simulink model "ACCMPC"  (R2023b)
settings: Solver=FixedStepDiscrete  StartTime=0.0  StopTime=1800  FixedStep=0.005  MaxStep=0.005  RelTol=1e-3  EnableMultiTasking=on
InitFcn:
  | load('DrivingCycles/WLTC.mat')
  | load('DrivingCycles/Mappa_Throttle.mat')
model workspace: external: MATLAB File C:\Users\stefa\Documents\EEPACC_MPC_CasADi_MATLAB\ACCMPC-ABO_CasADi\Init_ACCMPC_sim.m (data not in the file)
values from neighbouring files (symbols this model uses):
  OPTsettings = Settings(OPTsettings)    [Init_ACCMPC_sim.m]    (also in Main.m; Settings.m = GenerateUseCase(OPTsettings))
  V = SetVehicleParameters()    [Custom_plots.m]    (also in Init_ACCMPC_sfun.m; Init_ACCMPC_sim.m; Main.m; RunInit_ABMPC_sfun.m = SetParametersInternally())
undefined symbols (not defined in the file or in its folder): DiscIntNeverNeededParam, throttle_pedal, wheel_speed_radps, wheel_torque_Nm
libraries: slpidlib x4, simulink x1
(part 1 of 2)
settings Model: Creator=go  LastModifiedBy=stefa
settings SolverCC: ConcurrentTasks=on  AlgebraicLoopSolver=TrustRegion  PositivePriorityOrder=on  AutoInsertRateTranBlk=on
settings DataIOCC: SaveOutput=off  SaveTime=off  ReturnWorkspaceOutputs=off
settings OptimizationCC: DefaultParameterBehavior=Inlined  InlineInvariantSignals=on  EnhancedBackFolding=on  PassReuseOutputArgsAs=Individual arguments  StateBitsets=on  DataBitsets=on  ZeroExternalMemoryAtStartup=off  ZeroInternalMemoryAtStartup=off  NoFixptDivByZeroProtection=on  LifeSpan=1  OptimizeBlockOrder=speed  DifferentSizesBufferReuse=on  EfficientTunableParamExpr=on
settings DebuggingCC: TasksWithSamePriorityMsg=none  ParameterTunabilityLossMsg=error  UnconnectedInputMsg=warning  UnconnectedOutputMsg=warning  UnconnectedLineMsg=warning  ArithmeticOperatorsInVariantConditions=warning
settings HardwareCC: ProdBitPerPointer=32  ProdBitPerSizeT=32  ProdBitPerPtrDiffT=32  ProdLargestAtomicFloat=None  ProdIntDivRoundTo=Floor  ProdWordSize=32  ProdHWDeviceType=Generic->Custom
settings ModelReferenceCC: EnableRefExpFcnMdlSchedulingChecks=on
settings SFSimCC: SimUseLocalCustomCode=off  CustomCodeUndefinedFunction=UseInterfaceOnly  SimTargetLang=C++
settings RTWCC: Description=Embedded Coder  SystemTargetFile=ert.tlc  TLCOptions=-p0  GenCodeOnly=on  TemplateMakefile=ert_default_tmf  GenerateReport=on  RTWVerbose=off  RTWUseLocalCustomCode=off  Toolchain=Simulink Real-Time Toolchain  BuildConfiguration=Faster Runs  IncludeHyperlinkInReport=on  LaunchReport=on  CodeExecutionProfiling=on  TargetLang=C++  DLArmComputeVersion=19.05
settings CodeAppCC: ForceParamTrailComments=on  IgnoreCustomStorageClasses=off  MaxIdLength=95  OperatorAnnotations=on  SimulinkDataObjDesc=on  SFDataObjDesc=on  CustomSymbolStrGlobalVar=rt$N$M  CustomSymbolStrType=$N$M  CustomSymbolStrFcn=$N$M$F  CustomSymbolStrMacro=$N$M  InsertBlockDesc=on
settings ERTTargetCC: TargetLangStandard=C++03 (ISO)  CodeReplacementLibrary=ISO_C  GenerateSampleERTMain=on  SuppressErrorStatus=on  SupportAbsoluteTime=off  PurelyIntegerCode=on  SupportNonFinite=off  SupportComplex=off  InlinedParameterPlacement=NonHierarchical  RootIOFormat=Structure reference  ERTCustomFileTemplate=example_file_process.tlc

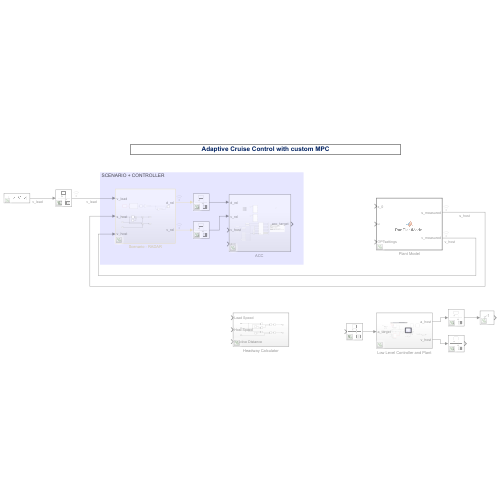
[thumbnail: Simulink's stored preview of the top-level diagram]
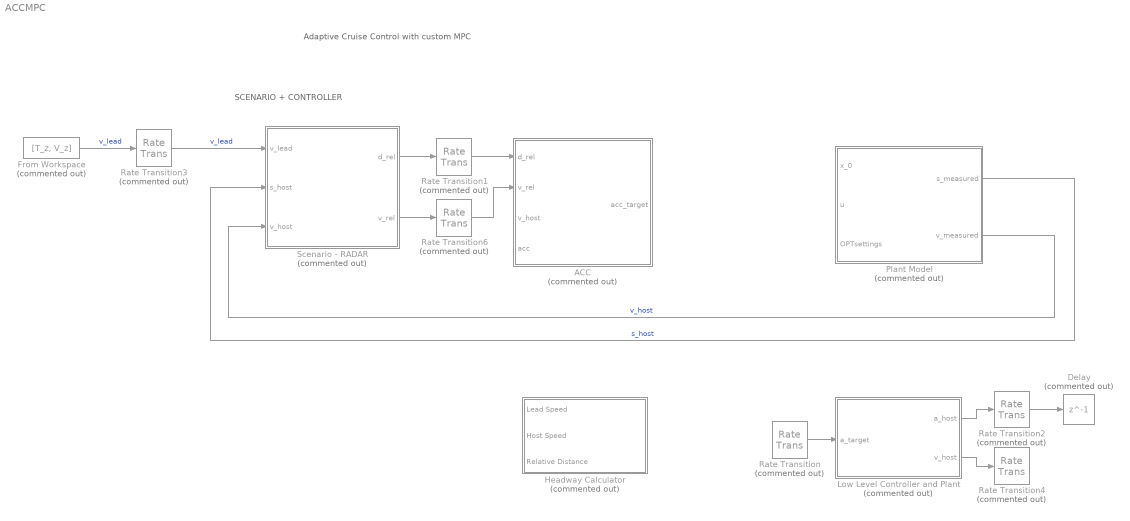
== system ACCMPC ==
  note: SCENARIO + CONTROLLER
  note: Adaptive Cruise Control with custom MPC
  "ACC " : Subsystem  Commented=on
  Delay : Delay  Commented=on  DelayLength=1
  From Workspace : FromWorkspace  Commented=on  VariableName=[T_z, V_z]  OutDataTypeStr=double  SampleTime=1
  Headway Calculator : Subsystem  Commented=on
  Low Level Controller and Plant : Subsystem  Commented=on
  Plant Model : MATLAB Function  Commented=on  TreatAsAtomicUnit=on
  Rate Transition : RateTransition  Commented=on  Integrity=off  Deterministic=off  OutPortSampleTime=0.005
  Rate Transition1 : RateTransition  Commented=on  OutPortSampleTime=0.2
  Rate Transition2 : RateTransition  Commented=on  Integrity=off  Deterministic=off  OutPortSampleTime=0.2
  Rate Transition3 : RateTransition  Commented=on  Integrity=off
  Rate Transition4 : RateTransition  Commented=on  Integrity=off  Deterministic=off  OutPortSampleTime=0.2
  Rate Transition6 : RateTransition  Commented=on  OutPortSampleTime=0.2
  Scenario - RADAR : Subsystem  Commented=on
  wires:
  Scenario - RADAR/1(d_rel) -> Rate Transition1/1
  Scenario - RADAR/2(v_rel) -> Rate Transition6/1
  Rate Transition/1 -> Low Level Controller and Plant/1(a_target)
  From Workspace/1 -> Rate Transition3/1  "v_lead"
  Rate Transition3/1 -> Scenario - RADAR/1(v_lead)  "v_lead"
  Low Level Controller and Plant/2(v_host) -> Rate Transition4/1
  Rate Transition1/1 -> "ACC "/1(d_rel)
  Rate Transition6/1 -> "ACC "/2(v_rel)
  Low Level Controller and Plant/1(a_host) -> Rate Transition2/1
  Rate Transition2/1 -> Delay/1
  Plant Model/2(v_measured) -> Scenario - RADAR/3(v_host)  "v_host"
  Plant Model/1(s_measured) -> Scenario - RADAR/2(s_host)  "s_host"

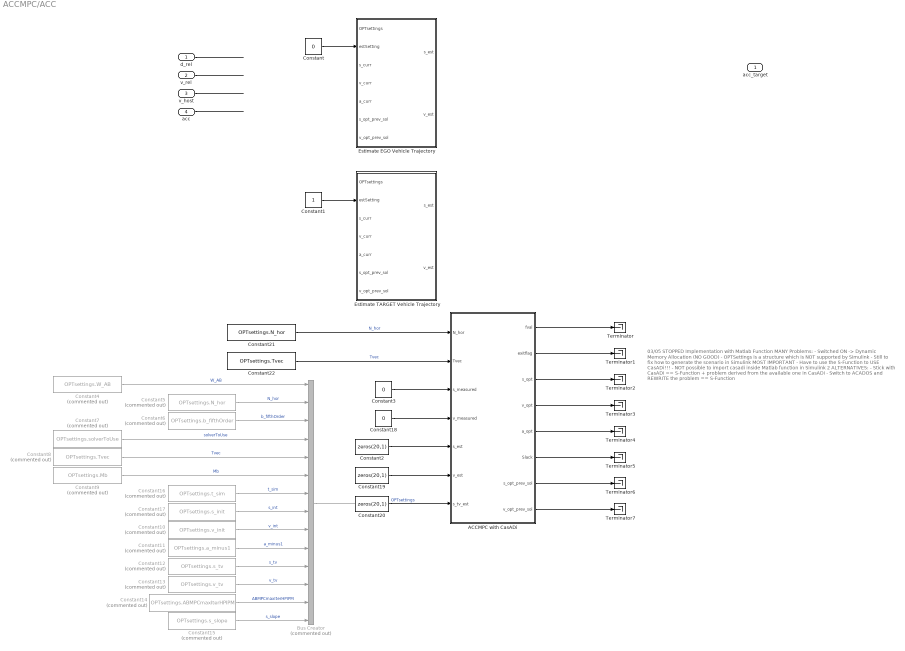
== system ACCMPC/ACC  ==
  note: 03/05 STOPPED Implementation with Matlab Function
      |
      | MANY Problems:
      | - Switched ON -> Dynamic Memory Allocation (NO GOOD)
      | - OPTSettings is a structure which is NOT supported by Simulink
      | - Still to fix how to generate the scenario in Simulink
      |
      | MOST IMPORTANT
      | - Have to use the S-Function to USE CasADi!!!
      | - NOT possible to import casadi inside Matlab function in Simulink
      |
      | 2 ALTERNATIVES:
      | - Stick with CasADi == S-Function + problem derived from the available one in CasADi
      | - Switch to ACADOS and REWRITE the problem == S-Function
  d_rel : Inport
  v_rel : Inport  Port=2
  v_host : Inport  Port=3
  acc : Inport  Port=4
  ACCMPC with CasADi : MATLAB Function  TreatAsAtomicUnit=on
  Bus Creator : BusCreator  Commented=on  Inputs=14
  Constant : Constant  Value=0
  Constant1 : Constant
  Constant10 : Constant  Commented=on  Value=OPTsettings.v_init
  Constant11 : Constant  Commented=on  Value=OPTsettings.a_minus1
  Constant12 : Constant  Commented=on  Value=OPTsettings.s_tv  VectorParams1D=off  OutDataTypeStr=double
  Constant13 : Constant  Commented=on  Value=OPTsettings.v_tv  VectorParams1D=off
  Constant14 : Constant  Commented=on  Value=OPTsettings.ABMPCmaxIterHPIPM
  Constant15 : Constant  Commented=on  Value=OPTsettings.s_slope  VectorParams1D=off
  Constant16 : Constant  Commented=on  Value=OPTsettings.t_sim
  Constant17 : Constant  Commented=on  Value=OPTsettings.s_init
  Constant18 : Constant  Value=0
  Constant19 : Constant  Value=zeros(20,1)
  Constant2 : Constant  Value=zeros(20,1)
  Constant20 : Constant  Value=zeros(20,1)
  Constant21 : Constant  Value=OPTsettings.N_hor
  Constant22 : Constant  Value=OPTsettings.Tvec  VectorParams1D=off
  Constant3 : Constant  Value=0
  Constant4 : Constant  Commented=on  Value=OPTsettings.W_AB  VectorParams1D=off
  Constant5 : Constant  Commented=on  Value=OPTsettings.N_hor
  Constant6 : Constant  Commented=on  Value=OPTsettings.b_fifthOrder  VectorParams1D=off
  Constant7 : Constant  Commented=on  Value=OPTsettings.solverToUse
  Constant8 : Constant  Commented=on  Value=OPTsettings.Tvec  VectorParams1D=off
  Constant9 : Constant  Commented=on  Value=OPTsettings.Mb  VectorParams1D=off
  Estimate EGO Vehicle Trajectory : MATLAB Function  TreatAsAtomicUnit=on
  Estimate TARGET Vehicle Trajectory : MATLAB Function  TreatAsAtomicUnit=on
  Terminator{,1..7} (8 alike) : Terminator
  "acc_target " : Outport
  wires:
  d_rel/1 -> ?
  v_rel/1 -> ?
  v_host/1 -> ?
  acc/1 -> ?
  Constant1/1 -> Estimate TARGET Vehicle Trajectory/2(estSetting)
  Constant/1 -> Estimate EGO Vehicle Trajectory/2(estSetting)
  Bus Creator/1 -> ?  "OPTsettings"
  Constant12/1 -> Bus Creator/11  "s_tv"
  Constant15/1 -> Bus Creator/14  "s_slope"
  Constant4/1 -> Bus Creator/1  "W_AB"
  Constant17/1 -> Bus Creator/8  "s_int"
  Constant10/1 -> Bus Creator/9  "v_int"
  Constant6/1 -> Bus Creator/3  "b_fifthOrder"
  Constant5/1 -> Bus Creator/2  "N_hor"
  Constant11/1 -> Bus Creator/10  "a_minus1"
  Constant14/1 -> Bus Creator/13  "ABMPCmaxIterHPIPM"
  Constant16/1 -> Bus Creator/7  "t_sim"
  Constant7/1 -> Bus Creator/4  "solverToUse"
  Constant8/1 -> Bus Creator/5  "Tvec"
  Constant13/1 -> Bus Creator/12  "v_tv"
  Constant9/1 -> Bus Creator/6  "Mb"
  Constant2/1 -> ACCMPC with CasADi/5(s_est)
  ACCMPC with CasADi/3(s_opt) -> Terminator2/1
  ACCMPC with CasADi/1(fval) -> Terminator/1
  Constant22/1 -> ACCMPC with CasADi/2(Tvec)  "Tvec"
  Constant20/1 -> ACCMPC with CasADi/7(s_tv_est)
  Constant21/1 -> ACCMPC with CasADi/1(N_hor)  "N_hor"
  ACCMPC with CasADi/4(v_opt) -> Terminator3/1
  Constant19/1 -> ACCMPC with CasADi/6(v_est)
  ACCMPC with CasADi/8(v_opt_prev_sol) -> Terminator7/1
  ACCMPC with CasADi/7(s_opt_prev_sol) -> Terminator6/1
  Constant18/1 -> ACCMPC with CasADi/4(v_measured)
  ACCMPC with CasADi/5(a_opt) -> Terminator4/1
  ACCMPC with CasADi/6(Slack) -> Terminator5/1
  ACCMPC with CasADi/2(exitflag) -> Terminator1/1
  Constant3/1 -> ACCMPC with CasADi/3(s_measured)

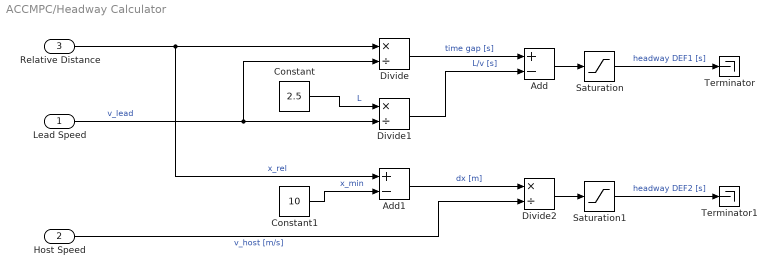
== system ACCMPC/Headway Calculator ==
  Lead Speed : Inport
  Host Speed : Inport  Port=2
  Relative Distance : Inport  Port=3
  Add : Sum  Inputs=+-
  Add1 : Sum  Inputs=+-
  Constant : Constant  Value=2.5
  Constant1 : Constant  Value=10
  Divide : Product  Inputs=*/
  Divide1 : Product  Inputs=*/
  Divide2 : Product  Inputs=*/
  Saturation : Saturate  UpperLimit=40  LowerLimit=0
  Saturation1 : Saturate  UpperLimit=40  LowerLimit=0
  Terminator : Terminator
  Terminator1 : Terminator
  wires:
  Lead Speed/1 -> Divide/2, Divide1/2  "v_lead"
  Constant/1 -> Divide1/1  "L"
  Divide1/1 -> Add/2  "L/v [s]"
  Saturation/1 -> Terminator/1  "headway DEF1 [s]"
  Relative Distance/1 -> Add1/1, Divide/1  "x_rel"
  Divide/1 -> Add/1  "time gap [s]"
  Constant1/1 -> Add1/2  "x_min"
  Add1/1 -> Divide2/1  "dx [m]"
  Host Speed/1 -> Divide2/2  "v_host [m/s]"
  Saturation1/1 -> Terminator1/1  "headway DEF2 [s]"
  Add/1 -> Saturation/1
  Divide2/1 -> Saturation1/1

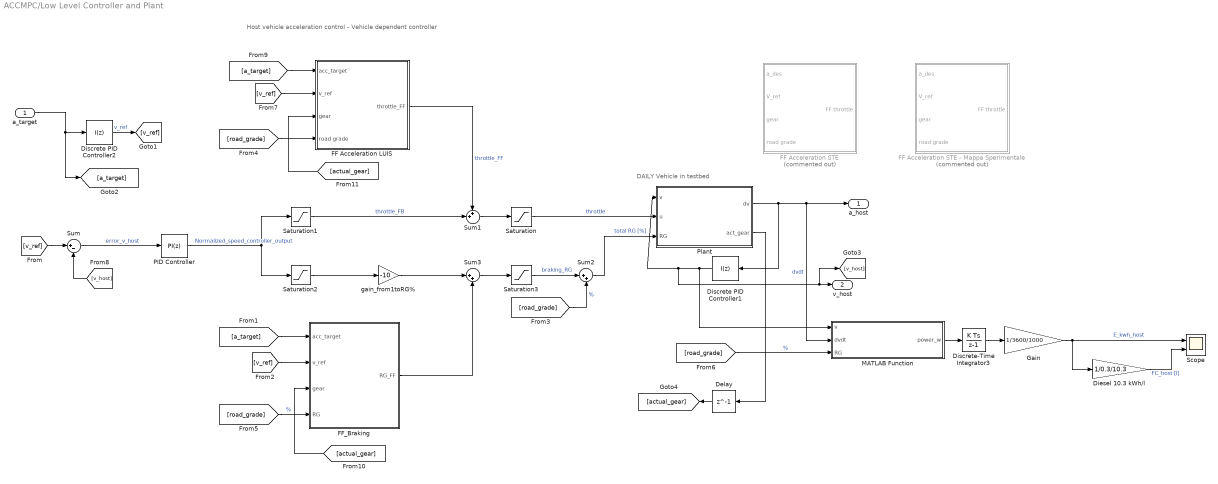
== system ACCMPC/Low Level Controller and Plant ==
  note: DAILY Vehicle in testbed
  note: Host vehicle acceleration control - Vehicle dependent controller
  a_target : Inport
  Delay : Delay  DelayLength=1  InitialCondition=1
  Diesel 10.3 kWh/l : Gain  Gain=1/0.3/10.3
  Discrete PID Controller1 : slpidlib/PID Controller  Controller=I  Form=Parallel  TimeDomain=Discrete-time  UseExternalTs=off  SampleTime=-1  IntegratorMethod=Forward Euler  FilterMethod=Forward Euler  ControllerParametersSource=internal  P=0  I=1  UseKiTs=off  D=0  N=100  UseFilter=on  TunerSelectOption=Transfer Function Based (PID Tuner App)  InitialConditionSource=internal  InitialConditionForIntegrator=0  InitialConditionForFilter=0  DifferentiatorICPrevScaledInput=0  ExternalReset=none  TrackingMode=off  Kt=1  LimitOutput=on  SatLimitsSource=internal  UpperSaturationLimit=inf  LowerSaturationLimit=0  LinearizeAsGain=off  AntiWindupMode=clamping  Kb=1  LimitIntegrator=off  UpperIntegratorSaturationLimit=inf  LowerIntegratorSaturationLimit=-inf  POutMin=[]  POutMax=[]  IOutMin=[]  IOutMax=[]  DOutMin=[]  DOutMax=[]  NOutMin=[]  NOutMax=[]  SumOutMin=[]  SumOutMax=[]  SaturationOutMin=[]  SaturationOutMax=[]  PParamMin=[]  PParamMax=[]  IParamMin=[]  IParamMax=[]  DParamMin=[]  DParamMax=[]  NParamMin=[]  NParamMax=[]  KbParamMin=[]  KbParamMax=[]  KtParamMin=[]  KtParamMax=[]  KbOutMin=[]  KbOutMax=[]  KtOutMin=[]  KtOutMax=[]  IntegratorOutMin=[]  IntegratorOutMax=[]  FilterOutMin=[]  FilterOutMax=[]  SumI1OutMin=[]  SumI1OutMax=[]  SumI2OutMin=[]  SumI2OutMax=[]  SumI3OutMin=[]  SumI3OutMax=[]  SumI4OutMin=[]  SumI4OutMax=[]  SumDOutMin=[]  SumDOutMax=[]  DifferentiatorOutMin=[]  DifferentiatorOutMax=[]  FilterDiffOutCoefMin=[]  FilterDiffOutCoefMax=[]  ReciprocalOutMin=[]  ReciprocalOutMax=[]  SumDenOutMin=[]  SumDenOutMax=[]  SumNumOutMin=[]  SumNumOutMax=[]  DivideOutMin=[]  DivideOutMax=[]  UdiffTsProdOutMin=[]  UdiffTsProdOutMax=[]  NTsProdOutMin=[]  NTsProdOutMax=[]  UintegralTsProdOutMin=[]  UintegralTsProdOutMax=[]  UngainTsProdOutMin=[]  UngainTsProdOutMax=[]  ClampingZeroOutDataTypeStr=Inherit: Inherit via back propagation  ClampingZeroOutMin=[]  ClampingZeroOutMax=[]  FilterDenConstantOutDataTypeStr=Inherit: Inherit via back propagation  FilterDenConstantOutMin=[]  FilterDenConstantOutMax=[]  PCopyOutDataTypeStr=Inherit: Inherit via back propagation  PCopyOutMin=[]  PCopyOutMax=[]  NCopyOutDataTypeStr=Inherit: Inherit via back propagation  NCopyOutMin=[]  NCopyOutMax=[]  IntegratorContinuousStateAttributes=''  IntegratorStateMustResolveToSignalObject=off  IntegratorRTWStateStorageClass=Auto  FilterContinuousStateAttributes=''  FilterStateMustResolveToSignalObject=off  FilterRTWStateStorageClass=Auto  ParallelPVariant=Disabled  IdealPVariant=Disabled  IVariant=InternalParameters  DVariant=Disabled  IntegratorVariant=Discrete  SatVariant=Enabled  AWVariant=DiscClampingParallel  PCopyVariant=Disabled  TRVariant=Disabled  FdbkBlocksVariant=Forward  IdealPFdbkVariant=Disabled  SatFdbkVariant=Disabled  DerivativeFilterVariant=Disabled  NVariant=Disabled  NCopyVariant=Disabled_SignalSpec  FilterICVariant=Disabled  IntegratorICVariant=InternalICs  ExternalResetVariant=Disabled  TRSumVariant=Passthrough  SumFdbkVariant=Disabled  SumVariant=Passthrough_I  TsampFilterVariant=InternalTs  TsampNgainVariant=Passthrough  TsampIntegralVariant=Disabled_SignalSpec  ExternalSaturationOutDataTypeStr=Inherit: Same as second input
  Discrete PID Controller2 : slpidlib/PID Controller  Controller=I  Form=Parallel  TimeDomain=Discrete-time  UseExternalTs=off  SampleTime=-1  IntegratorMethod=Forward Euler  FilterMethod=Forward Euler  ControllerParametersSource=internal  P=0  I=1  UseKiTs=off  D=0  N=100  UseFilter=on  TunerSelectOption=Transfer Function Based (PID Tuner App)  InitialConditionSource=internal  InitialConditionForIntegrator=0  InitialConditionForFilter=0  DifferentiatorICPrevScaledInput=0  ExternalReset=none  TrackingMode=off  Kt=1  LimitOutput=on  SatLimitsSource=internal  UpperSaturationLimit=inf  LowerSaturationLimit=0  LinearizeAsGain=off  AntiWindupMode=clamping  Kb=1  LimitIntegrator=off  UpperIntegratorSaturationLimit=inf  LowerIntegratorSaturationLimit=-inf  POutMin=[]  POutMax=[]  IOutMin=[]  IOutMax=[]  DOutMin=[]  DOutMax=[]  NOutMin=[]  NOutMax=[]  SumOutMin=[]  SumOutMax=[]  SaturationOutMin=[]  SaturationOutMax=[]  PParamMin=[]  PParamMax=[]  IParamMin=[]  IParamMax=[]  DParamMin=[]  DParamMax=[]  NParamMin=[]  NParamMax=[]  KbParamMin=[]  KbParamMax=[]  KtParamMin=[]  KtParamMax=[]  KbOutMin=[]  KbOutMax=[]  KtOutMin=[]  KtOutMax=[]  IntegratorOutMin=[]  IntegratorOutMax=[]  FilterOutMin=[]  FilterOutMax=[]  SumI1OutMin=[]  SumI1OutMax=[]  SumI2OutMin=[]  SumI2OutMax=[]  SumI3OutMin=[]  SumI3OutMax=[]  SumI4OutMin=[]  SumI4OutMax=[]  SumDOutMin=[]  SumDOutMax=[]  DifferentiatorOutMin=[]  DifferentiatorOutMax=[]  FilterDiffOutCoefMin=[]  FilterDiffOutCoefMax=[]  ReciprocalOutMin=[]  ReciprocalOutMax=[]  SumDenOutMin=[]  SumDenOutMax=[]  SumNumOutMin=[]  SumNumOutMax=[]  DivideOutMin=[]  DivideOutMax=[]  UdiffTsProdOutMin=[]  UdiffTsProdOutMax=[]  NTsProdOutMin=[]  NTsProdOutMax=[]  UintegralTsProdOutMin=[]  UintegralTsProdOutMax=[]  UngainTsProdOutMin=[]  UngainTsProdOutMax=[]  ClampingZeroOutDataTypeStr=Inherit: Inherit via back propagation  ClampingZeroOutMin=[]  ClampingZeroOutMax=[]  FilterDenConstantOutDataTypeStr=Inherit: Inherit via back propagation  FilterDenConstantOutMin=[]  FilterDenConstantOutMax=[]  PCopyOutDataTypeStr=Inherit: Inherit via back propagation  PCopyOutMin=[]  PCopyOutMax=[]  NCopyOutDataTypeStr=Inherit: Inherit via back propagation  NCopyOutMin=[]  NCopyOutMax=[]  IntegratorContinuousStateAttributes=''  IntegratorStateMustResolveToSignalObject=off  IntegratorRTWStateStorageClass=Auto  FilterContinuousStateAttributes=''  FilterStateMustResolveToSignalObject=off  FilterRTWStateStorageClass=Auto  ParallelPVariant=Disabled  IdealPVariant=Disabled  IVariant=InternalParameters  DVariant=Disabled  IntegratorVariant=Discrete  SatVariant=Enabled  AWVariant=DiscClampingParallel  PCopyVariant=Disabled  TRVariant=Disabled  FdbkBlocksVariant=Forward  IdealPFdbkVariant=Disabled  SatFdbkVariant=Disabled  DerivativeFilterVariant=Disabled  NVariant=Disabled  NCopyVariant=Disabled_SignalSpec  FilterICVariant=Disabled  IntegratorICVariant=InternalICs  ExternalResetVariant=Disabled  TRSumVariant=Passthrough  SumFdbkVariant=Disabled  SumVariant=Passthrough_I  TsampFilterVariant=InternalTs  TsampNgainVariant=Passthrough  TsampIntegralVariant=Disabled_SignalSpec  ExternalSaturationOutDataTypeStr=Inherit: Same as second input
  Discrete-Time Integrator3 : DiscreteIntegrator  SampleTime=-1  ICPrevOutput=DiscIntNeverNeededParam  ICPrevScaledInput=DiscIntNeverNeededParam
  FF Acceleration LUIS : Subsystem
  FF Acceleration STE : Subsystem  Commented=on
  FF Acceleration STE - Mappa Sperimentale : Subsystem  Commented=on
  FF_Braking : Subsystem
  Gain : Gain  Gain=1/3600/1000
  MATLAB Function : MATLAB Function  TreatAsAtomicUnit=on
  PID Controller : slpidlib/PID Controller  Controller=PI  Form=Parallel  TimeDomain=Discrete-time  UseExternalTs=off  SampleTime=-1  IntegratorMethod=Forward Euler  FilterMethod=Forward Euler  ControllerParametersSource=internal  P=0.54  I=0.54/16.67  UseKiTs=off  D=0  N=100  UseFilter=on  TunerSelectOption=Transfer Function Based (PID Tuner App)  InitialConditionSource=internal  InitialConditionForIntegrator=0  InitialConditionForFilter=0  DifferentiatorICPrevScaledInput=0  ExternalReset=none  TrackingMode=off  Kt=1  LimitOutput=on  SatLimitsSource=internal  UpperSaturationLimit=1  LowerSaturationLimit=-1  LinearizeAsGain=on  AntiWindupMode=clamping  Kb=1  LimitIntegrator=off  UpperIntegratorSaturationLimit=inf  LowerIntegratorSaturationLimit=-inf  POutMin=[]  POutMax=[]  IOutMin=[]  IOutMax=[]  DOutMin=[]  DOutMax=[]  NOutMin=[]  NOutMax=[]  SumOutMin=[]  SumOutMax=[]  SaturationOutMin=[]  SaturationOutMax=[]  PParamMin=[]  PParamMax=[]  IParamMin=[]  IParamMax=[]  DParamMin=[]  DParamMax=[]  NParamMin=[]  NParamMax=[]  KbParamMin=[]  KbParamMax=[]  KtParamMin=[]  KtParamMax=[]  KbOutMin=[]  KbOutMax=[]  KtOutMin=[]  KtOutMax=[]  IntegratorOutMin=[]  IntegratorOutMax=[]  FilterOutMin=[]  FilterOutMax=[]  SumI1OutMin=[]  SumI1OutMax=[]  SumI2OutMin=[]  SumI2OutMax=[]  SumI3OutMin=[]  SumI3OutMax=[]  SumI4OutMin=[]  SumI4OutMax=[]  SumDOutMin=[]  SumDOutMax=[]  DifferentiatorOutMin=[]  DifferentiatorOutMax=[]  FilterDiffOutCoefMin=[]  FilterDiffOutCoefMax=[]  ReciprocalOutMin=[]  ReciprocalOutMax=[]  SumDenOutMin=[]  SumDenOutMax=[]  SumNumOutMin=[]  SumNumOutMax=[]  DivideOutMin=[]  DivideOutMax=[]  UdiffTsProdOutMin=[]  UdiffTsProdOutMax=[]  NTsProdOutMin=[]  NTsProdOutMax=[]  UintegralTsProdOutMin=[]  UintegralTsProdOutMax=[]  UngainTsProdOutMin=[]  UngainTsProdOutMax=[]  ClampingZeroOutDataTypeStr=Inherit: Inherit via back propagation  ClampingZeroOutMin=[]  ClampingZeroOutMax=[]  FilterDenConstantOutDataTypeStr=Inherit: Inherit via back propagation  FilterDenConstantOutMin=[]  FilterDenConstantOutMax=[]  PCopyOutDataTypeStr=Inherit: Inherit via back propagation  PCopyOutMin=[]  PCopyOutMax=[]  NCopyOutDataTypeStr=Inherit: Inherit via back propagation  NCopyOutMin=[]  NCopyOutMax=[]  IntegratorContinuousStateAttributes=''  IntegratorStateMustResolveToSignalObject=off  IntegratorRTWStateStorageClass=Auto  FilterContinuousStateAttributes=''  FilterStateMustResolveToSignalObject=off  FilterRTWStateStorageClass=Auto  ParallelPVariant=InternalParameters  IdealPVariant=Disabled  IVariant=InternalParameters  DVariant=Disabled  IntegratorVariant=Discrete  SatVariant=Enabled  AWVariant=DiscClampingParallel  PCopyVariant=Disabled  TRVariant=Disabled  FdbkBlocksVariant=Forward  IdealPFdbkVariant=Disabled  SatFdbkVariant=Disabled  DerivativeFilterVariant=Disabled  NVariant=Disabled  NCopyVariant=Disabled_SignalSpec  FilterICVariant=Disabled  IntegratorICVariant=InternalICs  ExternalResetVariant=Disabled  TRSumVariant=Passthrough  SumFdbkVariant=Disabled  SumVariant=Sum_PI  TsampFilterVariant=InternalTs  TsampNgainVariant=Passthrough  TsampIntegralVariant=Disabled_SignalSpec  ExternalSaturationOutDataTypeStr=Inherit: Same as second input
  Plant : MATLAB Function  TreatAsAtomicUnit=on
  Saturation : Saturate  UpperLimit=1  LowerLimit=0
  Saturation1 : Saturate  UpperLimit=1  LowerLimit=0
  Saturation2 : Saturate  UpperLimit=0  LowerLimit=-1
  Saturation3 : Saturate  UpperLimit=100  LowerLimit=0
  Scope : Scope  NumInputPorts=2
  Sum : Sum  Inputs=|+-
  Sum1 : Sum  Inputs=++|
  Sum2 : Sum  Inputs=|++
  Sum3 : Sum  Inputs=|++
  gain_from1toRG% : Gain  Gain=-10
  a_host : Outport
  v_host : Outport  Port=2
  wires:
  Plant/1(dv) -> Discrete PID Controller1/1, MATLAB Function/2(dvdt), a_host/1  "dvdt"
  Discrete PID Controller1/1 -> MATLAB Function/1(v), [v_host], v_host/1, Plant/1(v)
  Sum1/1 -> Saturation/1
  Saturation1/1 -> Sum1/2  "throttle_FB"
  Plant/2(act_gear) -> Delay/1
  a_target/1 -> Discrete PID Controller2/1, [a_target]
  FF Acceleration LUIS/1(throttle_FF) -> Sum1/1  "throttle_FF"
  Discrete PID Controller2/1 -> [v_ref]  "v_ref"
  Saturation/1 -> Plant/2(u)  "throttle"
  [a_target] -> FF_Braking/1(acc_target)
  [v_ref] -> FF_Braking/2(v_ref)
  Sum2/1 -> Plant/3(RG)  "total RG [%]"
  [road_grade] -> Sum2/2  "%"
  [road_grade] -> FF Acceleration LUIS/4(road grade)
  [road_grade] -> FF_Braking/4(RG)  "%"
  MATLAB Function/1(power_w) -> Discrete-Time Integrator3/1
  [road_grade] -> MATLAB Function/3(RG)  "%"
  Gain/1 -> Diesel 10.3 kWh/l/1, Scope/1  "E_kwh_host"
  Discrete-Time Integrator3/1 -> Gain/1
  [v_host] -> Sum/2
  [v_ref] -> Sum/1
  Sum/1 -> PID Controller/1  "error_v_host"
  PID Controller/1 -> Saturation2/1, Saturation1/1  "Normalized_speed_controller_output"
  Saturation2/1 -> gain_from1toRG%/1
  gain_from1toRG%/1 -> Sum3/1
  FF_Braking/1(RG_FF) -> Sum3/2
  Sum3/1 -> Saturation3/1
  Saturation3/1 -> Sum2/1  "braking_RG"
  [v_ref] -> FF Acceleration LUIS/2(v_ref)
  [a_target] -> FF Acceleration LUIS/1(acc_target)
  Delay/1 -> [actual_gear]
  [actual_gear] -> FF_Braking/3(gear)
  [actual_gear] -> FF Acceleration LUIS/3(gear)
  Diesel 10.3 kWh/l/1 -> Scope/2  "FC_host [l]"

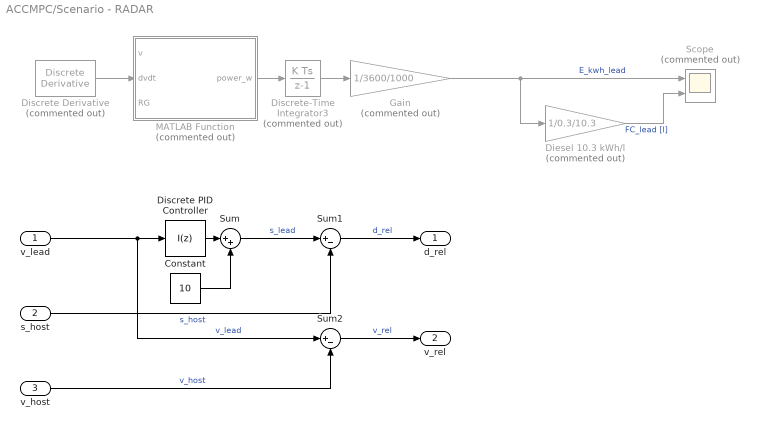
== system ACCMPC/Scenario - RADAR ==
  v_lead : Inport
  s_host : Inport  Port=2
  v_host : Inport  Port=3
  Constant : Constant  Value=10
  Diesel 10.3 kWh/l : Gain  Commented=on  Gain=1/0.3/10.3
  Discrete Derivative : simulink/Discrete/Discrete Derivative  Commented=on  gainval=1.0  ICPrevScaledInput=0.0  OutMin=[]  OutMax=[]  OutDataType=fixdt(1, 16)  OutScaling=2^-10  DoSatur=off
  Discrete PID Controller : slpidlib/PID Controller  Controller=I  Form=Parallel  TimeDomain=Discrete-time  UseExternalTs=off  SampleTime=-1  IntegratorMethod=Forward Euler  FilterMethod=Forward Euler  ControllerParametersSource=internal  P=0  I=1  UseKiTs=off  D=0  N=100  UseFilter=on  TunerSelectOption=Transfer Function Based (PID Tuner App)  InitialConditionSource=internal  InitialConditionForIntegrator=0  InitialConditionForFilter=0  DifferentiatorICPrevScaledInput=0  ExternalReset=none  TrackingMode=off  Kt=1  LimitOutput=off  SatLimitsSource=internal  UpperSaturationLimit=inf  LowerSaturationLimit=-inf  LinearizeAsGain=off  AntiWindupMode=none  Kb=1  LimitIntegrator=off  UpperIntegratorSaturationLimit=inf  LowerIntegratorSaturationLimit=-inf  POutMin=[]  POutMax=[]  IOutMin=[]  IOutMax=[]  DOutMin=[]  DOutMax=[]  NOutMin=[]  NOutMax=[]  SumOutMin=[]  SumOutMax=[]  SaturationOutMin=[]  SaturationOutMax=[]  PParamMin=[]  PParamMax=[]  IParamMin=[]  IParamMax=[]  DParamMin=[]  DParamMax=[]  NParamMin=[]  NParamMax=[]  KbParamMin=[]  KbParamMax=[]  KtParamMin=[]  KtParamMax=[]  KbOutMin=[]  KbOutMax=[]  KtOutMin=[]  KtOutMax=[]  IntegratorOutMin=[]  IntegratorOutMax=[]  FilterOutMin=[]  FilterOutMax=[]  SumI1OutMin=[]  SumI1OutMax=[]  SumI2OutMin=[]  SumI2OutMax=[]  SumI3OutMin=[]  SumI3OutMax=[]  SumI4OutMin=[]  SumI4OutMax=[]  SumDOutMin=[]  SumDOutMax=[]  DifferentiatorOutMin=[]  DifferentiatorOutMax=[]  FilterDiffOutCoefMin=[]  FilterDiffOutCoefMax=[]  ReciprocalOutMin=[]  ReciprocalOutMax=[]  SumDenOutMin=[]  SumDenOutMax=[]  SumNumOutMin=[]  SumNumOutMax=[]  DivideOutMin=[]  DivideOutMax=[]  UdiffTsProdOutMin=[]  UdiffTsProdOutMax=[]  NTsProdOutMin=[]  NTsProdOutMax=[]  UintegralTsProdOutMin=[]  UintegralTsProdOutMax=[]  UngainTsProdOutMin=[]  UngainTsProdOutMax=[]  ClampingZeroOutDataTypeStr=Inherit: Inherit via back propagation  ClampingZeroOutMin=[]  ClampingZeroOutMax=[]  FilterDenConstantOutDataTypeStr=Inherit: Inherit via back propagation  FilterDenConstantOutMin=[]  FilterDenConstantOutMax=[]  PCopyOutDataTypeStr=Inherit: Inherit via back propagation  PCopyOutMin=[]  PCopyOutMax=[]  NCopyOutDataTypeStr=Inherit: Inherit via back propagation  NCopyOutMin=[]  NCopyOutMax=[]  IntegratorContinuousStateAttributes=''  IntegratorStateMustResolveToSignalObject=off  IntegratorRTWStateStorageClass=Auto  FilterContinuousStateAttributes=''  FilterStateMustResolveToSignalObject=off  FilterRTWStateStorageClass=Auto  ParallelPVariant=Disabled  IdealPVariant=Disabled  IVariant=InternalParameters  DVariant=Disabled  IntegratorVariant=Discrete  SatVariant=Disabled  AWVariant=Passthrough  PCopyVariant=Disabled  TRVariant=Disabled  FdbkBlocksVariant=Forward  IdealPFdbkVariant=Disabled  SatFdbkVariant=Disabled  DerivativeFilterVariant=Disabled  NVariant=Disabled  NCopyVariant=Disabled_SignalSpec  FilterICVariant=Disabled  IntegratorICVariant=InternalICs  ExternalResetVariant=Disabled  TRSumVariant=Passthrough  SumFdbkVariant=Disabled  SumVariant=Passthrough_I  TsampFilterVariant=InternalTs  TsampNgainVariant=Passthrough  TsampIntegralVariant=Disabled_SignalSpec  ExternalSaturationOutDataTypeStr=Inherit: Same as second input
  Discrete-Time Integrator3 : DiscreteIntegrator  Commented=on  SampleTime=-1  ICPrevOutput=DiscIntNeverNeededParam  ICPrevScaledInput=DiscIntNeverNeededParam
  Gain : Gain  Commented=on  Gain=1/3600/1000
  MATLAB Function : MATLAB Function  Commented=on  TreatAsAtomicUnit=on
  Scope : Scope  Commented=on  NumInputPorts=2
  Sum : Sum  Inputs=|++
  Sum1 : Sum  Inputs=|+-
  Sum2 : Sum  Inputs=|+-
  d_rel : Outport
  v_rel : Outport  Port=2
  wires:
  Sum1/1 -> d_rel/1  "d_rel"
  Constant/1 -> Sum/2
  Discrete PID Controller/1 -> Sum/1
  Sum2/1 -> v_rel/1  "v_rel"
  s_host/1 -> Sum1/2  "s_host"
  Sum/1 -> Sum1/1  "s_lead"
  v_host/1 -> Sum2/2  "v_host"
  MATLAB Function/1(power_w) -> Discrete-Time Integrator3/1
  Discrete Derivative/1 -> MATLAB Function/2(dvdt)
  Gain/1 -> Diesel 10.3 kWh/l/1, Scope/1  "E_kwh_lead"
  Discrete-Time Integrator3/1 -> Gain/1
  v_lead/1 -> Sum2/1, Discrete PID Controller/1  "v_lead"
  Diesel 10.3 kWh/l/1 -> Scope/2  "FC_lead [l]"

== system ACCMPC/Low Level Controller and Plant/FF Acceleration LUIS ==
  acc_target : Inport
  v_ref : Inport  Port=2
  gear : Inport  Port=3
  road grade : Inport  Port=4
  FEEDFORWARD : MATLAB Function  TreatAsAtomicUnit=on
  throttle_FF : Outport
  wires:
  gear/1 -> FEEDFORWARD/4(gear)
  acc_target/1 -> FEEDFORWARD/1(acc_target)
  FEEDFORWARD/1(uff) -> throttle_FF/1  "throttle_FF"
  v_ref/1 -> FEEDFORWARD/2(v_ref)
  road grade/1 -> FEEDFORWARD/3(RG)

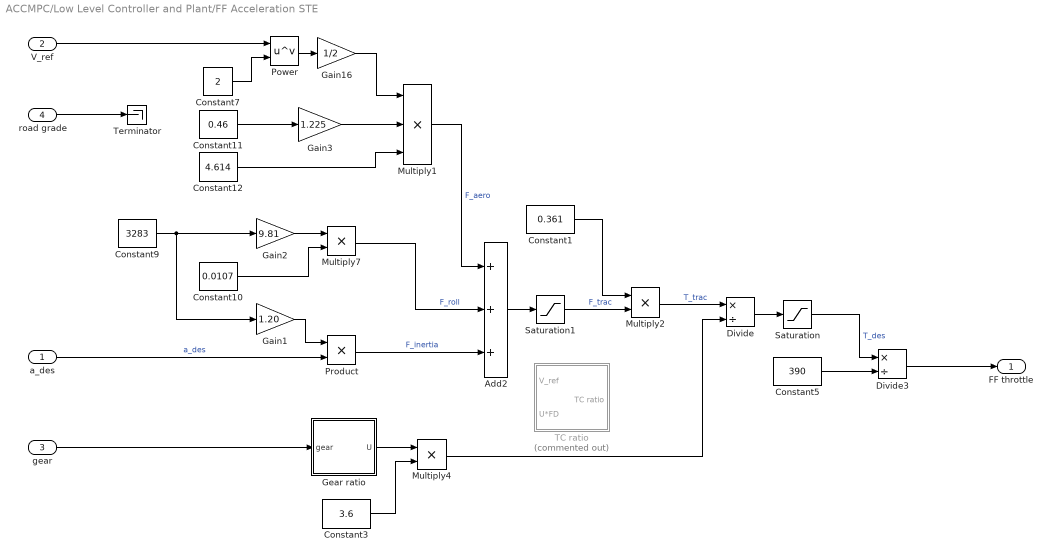
== system ACCMPC/Low Level Controller and Plant/FF Acceleration STE ==
  a_des : Inport
  V_ref : Inport  Port=2
  gear : Inport  Port=3
  road grade : Inport  Port=4
  Add2 : Sum  Inputs=+++
  Constant1 : Constant  Value=0.361
  Constant10 : Constant  Value=0.0107
  Constant11 : Constant  Value=0.46
  Constant12 : Constant  Value=4.614
  Constant3 : Constant  Value=3.6
  Constant5 : Constant  Value=390
  Constant7 : Constant  Value=2
  Constant9 : Constant  Value=3283
  Divide : Product  Inputs=*/
  Divide3 : Product  Inputs=*/
  Gain1 : Gain  Gain=1.20
  Gain16 : Gain  Gain=1/2
  Gain2 : Gain  Gain=9.81
  Gain3 : Gain  Gain=1.225
  Gear ratio : Subsystem
  Multiply1 : Product  Inputs=3
  Multiply2 : Product
  Multiply4 : Product
  Multiply7 : Product
  Power : Math  Operator=pow
  Product : Product
  Saturation : Saturate  UpperLimit=390  LowerLimit=0
  Saturation1 : Saturate  UpperLimit=inf  LowerLimit=0
  TC ratio : Subsystem  Commented=on
  Terminator : Terminator
  FF throttle : Outport
  wires:
  Multiply1/1 -> Add2/1  "F_aero"
  Gain16/1 -> Multiply1/1
  Gear ratio/1(U) -> Multiply4/1
  Constant3/1 -> Multiply4/2
  a_des/1 -> Product/2  "a_des"
  Constant9/1 -> Gain1/1, Gain2/1
  Constant11/1 -> Gain3/1
  Saturation/1 -> Divide3/1  "T_des"
  Add2/1 -> Saturation1/1
  Constant10/1 -> Multiply7/2
  Saturation1/1 -> Multiply2/2  "F_trac"
  Power/1 -> Gain16/1
  Multiply7/1 -> Add2/2  "F_roll"
  Gain2/1 -> Multiply7/1
  Constant7/1 -> Power/2
  Constant1/1 -> Multiply2/1
  Multiply2/1 -> Divide/1  "T_trac"
  Constant12/1 -> Multiply1/3
  Product/1 -> Add2/3  "F_inertia"
  Divide3/1 -> FF throttle/1
  Gain3/1 -> Multiply1/2
  Constant5/1 -> Divide3/2
  V_ref/1 -> Power/1
  Divide/1 -> Saturation/1
  Multiply4/1 -> Divide/2
  Gain1/1 -> Product/1
  gear/1 -> Gear ratio/1(gear)
  road grade/1 -> Terminator/1

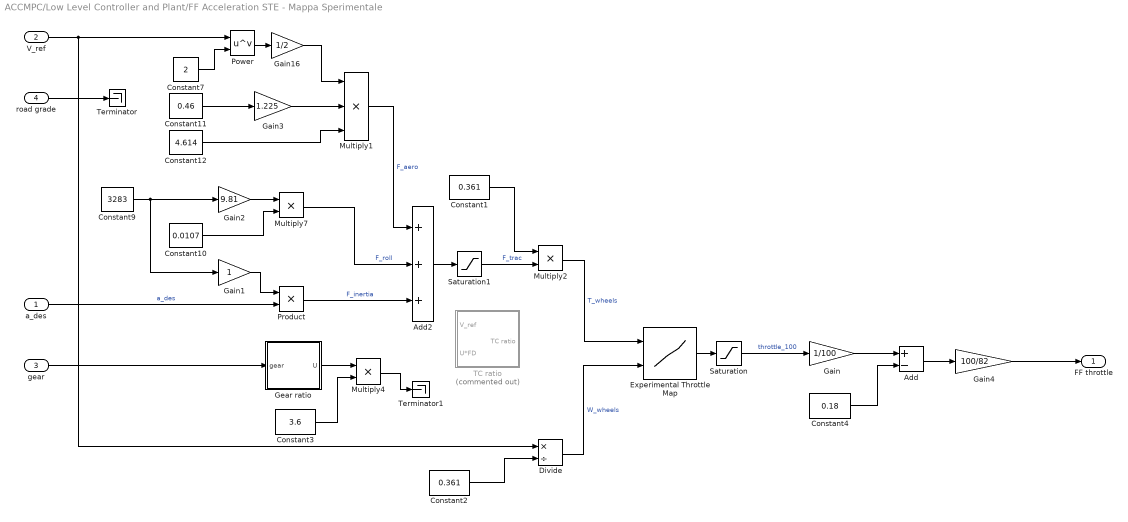
== system ACCMPC/Low Level Controller and Plant/FF Acceleration STE - Mappa Sperimentale ==
  a_des : Inport
  V_ref : Inport  Port=2
  gear : Inport  Port=3
  road grade : Inport  Port=4
  Add : Sum  Inputs=+-
  Add2 : Sum  Inputs=+++
  Constant1 : Constant  Value=0.361
  Constant10 : Constant  Value=0.0107
  Constant11 : Constant  Value=0.46
  Constant12 : Constant  Value=4.614
  Constant2 : Constant  Value=0.361
  Constant3 : Constant  Value=3.6
  Constant4 : Constant  Value=0.18
  Constant7 : Constant  Value=2
  Constant9 : Constant  Value=3283
  Divide : Product  Inputs=*/
  Experimental Throttle Map : Lookup_n-D  BreakpointsForDimension1=wheel_torque_Nm  BreakpointsForDimension2=wheel_speed_radps  Table=throttle_pedal  InternalRulePriority=Speed  RndMeth=Simplest
      settings: InputPortMap=u0,u1
  Gain : Gain  Gain=1/100
  Gain1 : Gain
  Gain16 : Gain  Gain=1/2
  Gain2 : Gain  Gain=9.81
  Gain3 : Gain  Gain=1.225
  Gain4 : Gain  Gain=100/82
  Gear ratio : Subsystem
  Multiply1 : Product  Inputs=3
  Multiply2 : Product
  Multiply4 : Product
  Multiply7 : Product
  Power : Math  Operator=pow
  Product : Product
  Saturation : Saturate  UpperLimit=100  LowerLimit=0
  Saturation1 : Saturate  UpperLimit=inf  LowerLimit=0
  TC ratio : Subsystem  Commented=on
  Terminator : Terminator
  Terminator1 : Terminator
  FF throttle : Outport
  wires:
  Multiply1/1 -> Add2/1  "F_aero"
  Gain16/1 -> Multiply1/1
  Gear ratio/1(U) -> Multiply4/1
  Constant3/1 -> Multiply4/2
  a_des/1 -> Product/2  "a_des"
  Constant9/1 -> Gain1/1, Gain2/1
  Constant11/1 -> Gain3/1
  Add2/1 -> Saturation1/1
  Constant10/1 -> Multiply7/2
  Saturation1/1 -> Multiply2/2  "F_trac"
  Power/1 -> Gain16/1
  Multiply7/1 -> Add2/2  "F_roll"
  Gain2/1 -> Multiply7/1
  Constant7/1 -> Power/2
  Constant1/1 -> Multiply2/1
  Constant12/1 -> Multiply1/3
  Product/1 -> Add2/3  "F_inertia"
  Gain3/1 -> Multiply1/2
  V_ref/1 -> Divide/1, Power/1
  Multiply4/1 -> Terminator1/1
  Gain1/1 -> Product/1
  gear/1 -> Gear ratio/1(gear)
  road grade/1 -> Terminator/1
  Constant2/1 -> Divide/2
  Multiply2/1 -> Experimental Throttle Map/1  "T_wheels"
  Divide/1 -> Experimental Throttle Map/2  "W_wheels"
  Experimental Throttle Map/1 -> Saturation/1
  Saturation/1 -> Gain/1  "throttle_100"
  Gain/1 -> Add/1
  Add/1 -> Gain4/1
  Constant4/1 -> Add/2
  Gain4/1 -> FF throttle/1

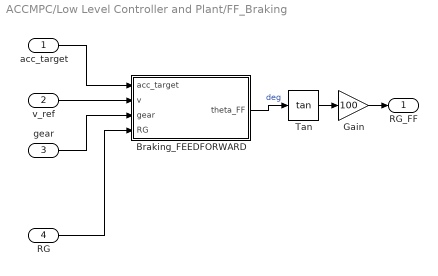
== system ACCMPC/Low Level Controller and Plant/FF_Braking ==
  acc_target : Inport
  v_ref : Inport  Port=2
  gear : Inport  Port=3
  RG : Inport  Port=4
  Braking_FEEDFORWARD : MATLAB Function  TreatAsAtomicUnit=on
  Gain : Gain  Gain=100
  Tan : Trigonometry  Operator=tan
  RG_FF : Outport
  wires:
  gear/1 -> Braking_FEEDFORWARD/3(gear)
  acc_target/1 -> Braking_FEEDFORWARD/1(acc_target)
  Braking_FEEDFORWARD/1(theta_FF) -> Tan/1  "deg"
  v_ref/1 -> Braking_FEEDFORWARD/2(v)
  Tan/1 -> Gain/1
  Gain/1 -> RG_FF/1
  RG/1 -> Braking_FEEDFORWARD/4(RG)

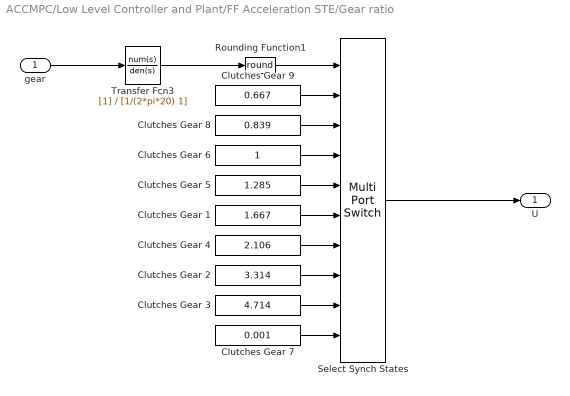
== system ACCMPC/Low Level Controller and Plant/FF Acceleration STE/Gear ratio ==
  gear : Inport
  Clutches Gear 1 : Constant  Value=1.667  SampleTime=0
  Clutches Gear 2 : Constant  Value=3.314  SampleTime=0
  Clutches Gear 3 : Constant  Value=4.714  SampleTime=0
  Clutches Gear 4 : Constant  Value=2.106  SampleTime=0
  Clutches Gear 5 : Constant  Value=1.285  SampleTime=0
  Clutches Gear 6 : Constant  SampleTime=0
  Clutches Gear 7 : Constant  Value=0.001  SampleTime=0
  Clutches Gear 8 : Constant  Value=0.839  SampleTime=0
  Clutches Gear 9 : Constant  Value=0.667  SampleTime=0
  Rounding Function1 : Rounding  Operator=round
  Select Synch States : MultiPortSwitch  DataPortOrder=Specify indices  DataPortIndices={8,7,6,5,4,3,2,1,0}  DiagnosticForDefault=None  SaturateOnIntegerOverflow=off  InputSameDT=off
  Transfer Fcn3 : TransferFcn  Denominator=[1/(2*pi*20) 1]
  U : Outport  VectorParamsAs1DForOutWhenUnconnected=off
  wires:
  gear/1 -> Transfer Fcn3/1
  Select Synch States/1 -> U/1
  Clutches Gear 1/1 -> Select Synch States/6
  Clutches Gear 2/1 -> Select Synch States/8
  Clutches Gear 6/1 -> Select Synch States/4
  Clutches Gear 5/1 -> Select Synch States/5
  Clutches Gear 4/1 -> Select Synch States/7
  Rounding Function1/1 -> Select Synch States/1
  Clutches Gear 7/1 -> Select Synch States/10
  Clutches Gear 9/1 -> Select Synch States/2
  Clutches Gear 8/1 -> Select Synch States/3
  Clutches Gear 3/1 -> Select Synch States/9
  Transfer Fcn3/1 -> Rounding Function1/1

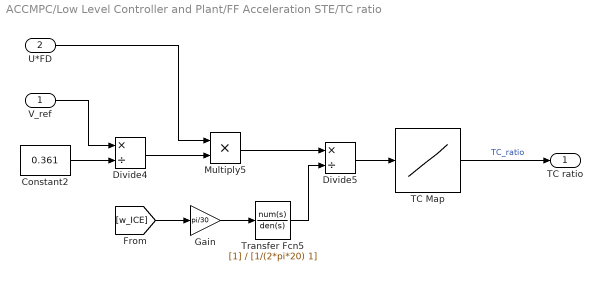
== system ACCMPC/Low Level Controller and Plant/FF Acceleration STE/TC ratio ==
  V_ref : Inport
  U*FD : Inport  Port=2
  Constant2 : Constant  Value=0.361
  Divide4 : Product  Inputs=*/
  Divide5 : Product  Inputs=*/
  Gain : Gain  Gain=pi/30
  Multiply5 : Product
  TC Map : Lookup_n-D  NumberOfTableDimensions=1  BreakpointsForDimension1=[0 0.50 0.60 0.70 0.80 0.87 0.92 0.94 0.96 0.97]  Table=[1.911 1.413 1.303 1.201 1.109 1.053 1.018 1.006 0.994 0.989]  InternalRulePriority=Speed  RndMeth=Simplest
  Transfer Fcn5 : TransferFcn  Denominator=[1/(2*pi*20) 1]
  TC ratio : Outport
  wires:
  Transfer Fcn5/1 -> Divide5/2
  Divide4/1 -> Multiply5/2
  Multiply5/1 -> Divide5/1
  Constant2/1 -> Divide4/2
  [w_ICE] -> Gain/1
  TC Map/1 -> TC ratio/1  "TC_ratio"
  Divide5/1 -> TC Map/1
  U*FD/1 -> Multiply5/1
  V_ref/1 -> Divide4/1
  Gain/1 -> Transfer Fcn5/1

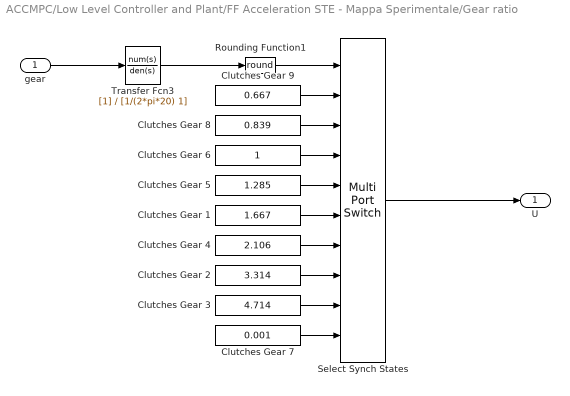
== system ACCMPC/Low Level Controller and Plant/FF Acceleration STE - Mappa Sperimentale/Gear ratio ==
  gear : Inport
  Clutches Gear 1 : Constant  Value=1.667  SampleTime=0
  Clutches Gear 2 : Constant  Value=3.314  SampleTime=0
  Clutches Gear 3 : Constant  Value=4.714  SampleTime=0
  Clutches Gear 4 : Constant  Value=2.106  SampleTime=0
  Clutches Gear 5 : Constant  Value=1.285  SampleTime=0
  Clutches Gear 6 : Constant  SampleTime=0
  Clutches Gear 7 : Constant  Value=0.001  SampleTime=0
  Clutches Gear 8 : Constant  Value=0.839  SampleTime=0
  Clutches Gear 9 : Constant  Value=0.667  SampleTime=0
  Rounding Function1 : Rounding  Operator=round
  Select Synch States : MultiPortSwitch  DataPortOrder=Specify indices  DataPortIndices={8,7,6,5,4,3,2,1,0}  DiagnosticForDefault=None  SaturateOnIntegerOverflow=off  InputSameDT=off
  Transfer Fcn3 : TransferFcn  Denominator=[1/(2*pi*20) 1]
  U : Outport  VectorParamsAs1DForOutWhenUnconnected=off
  wires:
  gear/1 -> Transfer Fcn3/1
  Select Synch States/1 -> U/1
  Clutches Gear 1/1 -> Select Synch States/6
  Clutches Gear 2/1 -> Select Synch States/8
  Clutches Gear 6/1 -> Select Synch States/4
  Clutches Gear 5/1 -> Select Synch States/5
  Clutches Gear 4/1 -> Select Synch States/7
  Rounding Function1/1 -> Select Synch States/1
  Clutches Gear 7/1 -> Select Synch States/10
  Clutches Gear 9/1 -> Select Synch States/2
  Clutches Gear 8/1 -> Select Synch States/3
  Clutches Gear 3/1 -> Select Synch States/9
  Transfer Fcn3/1 -> Rounding Function1/1

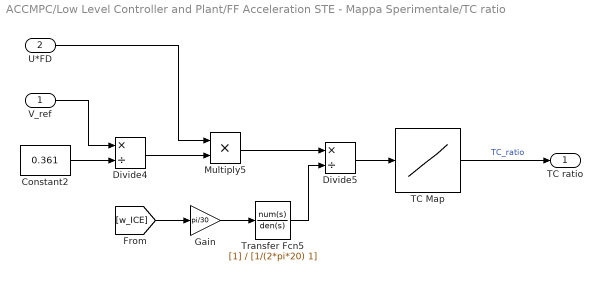
== system ACCMPC/Low Level Controller and Plant/FF Acceleration STE - Mappa Sperimentale/TC ratio ==
  V_ref : Inport
  U*FD : Inport  Port=2
  Constant2 : Constant  Value=0.361
  Divide4 : Product  Inputs=*/
  Divide5 : Product  Inputs=*/
  Gain : Gain  Gain=pi/30
  Multiply5 : Product
  TC Map : Lookup_n-D  NumberOfTableDimensions=1  BreakpointsForDimension1=[0 0.50 0.60 0.70 0.80 0.87 0.92 0.94 0.96 0.97]  Table=[1.911 1.413 1.303 1.201 1.109 1.053 1.018 1.006 0.994 0.989]  InternalRulePriority=Speed  RndMeth=Simplest
  Transfer Fcn5 : TransferFcn  Denominator=[1/(2*pi*20) 1]
  TC ratio : Outport
  wires:
  Transfer Fcn5/1 -> Divide5/2
  Divide4/1 -> Multiply5/2
  Multiply5/1 -> Divide5/1
  Constant2/1 -> Divide4/2
  [w_ICE] -> Gain/1
  TC Map/1 -> TC ratio/1  "TC_ratio"
  Divide5/1 -> TC Map/1
  U*FD/1 -> Multiply5/1
  V_ref/1 -> Divide4/1
  Gain/1 -> Transfer Fcn5/1

== matlab function ACCMPC/ACC /Estimate TARGET Vehicle Trajectory ==
  data: OPTsettings input; estSetting input; s_curr input; s_est output size=1; v_est output; v_curr input; a_curr input; s_opt_prev_sol input; v_opt_prev_sol input
function [s_est, v_est] = EstimateVehicleTrajectory(OPTsettings, estSetting, s_curr, v_curr, a_curr, s_opt_prev_sol, v_opt_prev_sol)
% EstimateVehicleTrajectory Estimates the trajectory of the target or ego vehicle along the prediction horizon
%
%   Inputs:
%       OPTsettings    : struct with settings for the optimization
%       estSetting     : (0) estimate ego vehicle trajectory for FBMPC or ABMPC; (1) estimate target vehicle trajectory; (2) estimation for the TVMPC; (3) estimation for the BLMPC
%       s_curr         : current travel distance for the estimate
%       v_curr         : current velocity for the estimate
%       a_curr         : current acceleration for the estimate
%       s_opt_prev_sol : optimal solution for the travel distance in the horizon of the previous QP
%       v_opt_prev_sol : optimal solution for the velocity in the horizon of the previous QP
%
%   Outputs:
%       s_est          : estimate of the travel distance along the horizon
%       v_est          : estimate of the velocity along the horizon
        
    %% initialization

    % extract settings
    if estSetting == 2
        % for TVMPC
        paramEstSetting = OPTsettings.TV_trajEstSett;
        Ts              = OPTsettings.TV_Ts;
        N_hor           = OPTsettings.TV_N_hor;
    elseif estSetting == 3
        % for BLMPC
        paramEstSetting = OPTsettings.BL_trajEstSett;
        Ts              = OPTsettings.BL_Ts;
        N_hor           = OPTsettings.BL_N_hor;
    else
        % for ABMPC and FBPMC
        N_hor = OPTsettings.N_hor;
        Tvec  = OPTsettings.Tvec;
        if estSetting == 0
            paramEstSetting = OPTsettings.paramEstSetting;
        else
            paramEstSetting = OPTsettings.TVestSetting;
        end
    end

    % const. acceleration time when using paramEstSetting 2
    if estSetting == 1
        tConstACC = OPTsettings.tConstACC_tar;
    else
        tConstACC = OPTsettings.tConstACC_ego;
    end

    % initialize arrays
    s_est = zeros(N_hor+1,1);
    v_est = zeros(N_hor+1,1);

    %% Estimation

    % Estimate distance and velocity for the full horizon
    if paramEstSetting == 0
        % constant velocity
        s_est(1) = s_curr;
        for i = 2:N_hor+1
            if estSetting < 2
                Ts = Tvec(i-1);
            end
            s_est(i) = s_est(i-1) + Ts*v_curr;
        end
        v_est = v_curr*ones(1,N_hor+1);
    elseif paramEstSetting == 1
        % constant acceleration
        s_est(1) = s_curr;
        v_est(1) = v_curr;
        for i = 2:N_hor+1
            if estSetting < 2
                Ts = Tvec(i-1);
            end
            if i <= tConstACC/Ts && v_est(i-1) + Ts*a_curr > 0
                v_est(i) = v_est(i-1) + Ts*a_curr;
            else
                v_est(i) = v_est(i-1);
            end
            s_est(i) = s_est(i-1) + Ts*v_est(i-1);
            
        end
    else
        if estSetting < 2
            Ts = Tvec(end);
        end
        % use the previous MPC solutions
        s_est = [s_curr; s_opt_prev_sol(3:end); s_opt_prev_sol(end)+Ts*v_opt_prev_sol(end)];
        v_est = [v_curr; v_opt_prev_sol(3:end); v_opt_prev_sol(end)];
    end

end

== matlab function ACCMPC/ACC /ACCMPC with CasADi ==
  data: N_hor input; Tvec input; fval output size=1; exitflag output; s_measured input; s_opt output; v_opt output; v_measured input; s_est input; v_est input; s_tv_est input; a_opt output; Slack output; s_opt_prev_sol output; v_opt_prev_sol output; OPTsettings parameter; V parameter
function [fval,exitflag,s_opt,v_opt,a_opt,Slack,s_opt_prev_sol,v_opt_prev_sol] = ACCMPC(N_hor, Tvec, s_measured,v_measured,s_est,v_est,s_tv_est,OPTsettings, V)
% ACCMPC Produces the MPC Control Action in closed loop
%
%   Inputs:
%       OPTsettings    : struct with settings for the optimization
%
%   Outputs:
%       tbd            : tbd

persistent H c G z_lb z_ub g_lb g_ub
% persistent W N_hor b_fifthOrder solverToUse Tvec Mb t_sim s_0 v_0 a_minus1
persistent t_0 n_x n_u n_x_u N a_minus1 Ts 
persistent options

    %% Unpack settings
    % OK with RunInit_ABMPC
    
    %% Initialize matrices and create solver
    % OK with RunInit_ABMPC

    % numbers of variables
    % qpOASES
    n_x = 2; % [s; v]
    n_u = 5; % [a; xi_v; xi_h; xi_s; xi_f]
    n_x_u = n_x + n_u;

    % initialization of matrices: estimated values don't matter
    % s_est       = ones(N_hor,1);
    % v_est       = ones(N_hor,1);
    % s_tv_est    = ones(N_hor,1);
    t_0         = 0;

    % Initialize other
    a_minus1    = 0;
    Ts = 0.5;
    N = N_hor;

    %% Formulate the the QP
    [H,c,G,z_lb,z_ub,g_lb,g_ub] = CreateQP_ABSimulink(OPTsettings,n_x,n_u,s_measured,v_measured,s_est,v_est,s_tv_est,t_0,a_minus1);

    %% Postprocessing

    % Delete zero rows in G
    zeroColsG = all(~G,2);
    G(zeroColsG,:) = [];
        
    % Fix lengths of bounds on G
    g_lb = g_lb(1:size(G,1));
    g_ub = g_ub(1:size(G,1));

    % Transform optimization matrices to dense versions
    % qpOASES
        % Create state space matrices
        A = zeros(N_hor,n_x,n_x);
        B = zeros(N_hor,n_x,n_u);
        D = zeros(N_hor,n_x);
        for k = 1:N_hor
            A(k,1:2,1:2) = [1, Tvec(k); 0, 1];
            B(k,1,1) = .5*Tvec(k)^2;
            B(k,2,1) = Tvec(k);
            D(k,:,:) = [0; 0];
        end
        % dense qpOASES
        [H,c,G,g_lb,g_ub,Psi,d] = TransformToDenseFormulation(N_hor,A,B,D,H,c,G,g_lb,g_ub,n_x,n_u,s_measured,v_measured);

    % % create problem structure and solver
    % % qpOASES
    % opts = struct;
    % opts.printLevel = 'low'; % options: none, low, medium, high, debug_iter, tabular
    % opts.error_on_fail = false;
    % prob = struct('h', SX(H).sparsity(), 'a', SX(G).sparsity());
    % QPsolver = conic('QPsolver','qpoases',prob,opts);
    
    %% Solve MPC and extract states and controls

    % solve the problem and extract the optimal solution
    % qpOASES in CasADi
    % sol = QPsolver('h',H,'g',c,'a',G,'lbx',z_lb,'ubx',z_ub,'lba',g_lb,'uba',g_ub);
    % optSol.exitMessage = ~QPsolver.stats().success;
    % optSol.solverTime = QPsolver.stats().t_proc_solver;
    % z_opt = full(sol.x);
    % % Transform dense z to sparse z to get the states as well
    % if solverToUse == 1
    %     z_opt = Psi*z_opt+d;
    % end
    % quadprog
    options = optimoptions('quadprog','Display','off','Algorithm','active-set');
    [z_opt,fval,exitflag,~,~]  = quadprog(H,c,[],[],[G;-G],[g_ub;-g_lb],z_lb,z_ub,zeros(N*n_x_u),options);
    % Transform dense z to sparse z to get the states as well
    z_opt = Psi*z_opt+d;

    % extract optimal state and control variables
    s_opt = z_opt(1);
    v_opt = z_opt(2);
    % qpOASES
        a_opt    = z_opt(3);     
        Slack = zeros(4,1);
        Slack(1,1) = z_opt(4);
        Slack(2,1) = z_opt(5);
        Slack(3,1) = z_opt(6);
        Slack(4,1) = z_opt(7);

    % save previous solution's trajectory for approximations in the next step
    s_opt_prev_sol = z_opt(1:n_x_u:end);
    v_opt_prev_sol = z_opt(2:n_x_u:end);

    %% determine required forces

    % get the estimated road angle
    % theta = InterpPWA(s_measured,OPTsettings.s_slope,OPTsettings.slope);
    theta = 0;

    % Total resistance force (sum of aerodynamic, rolling and grading resistance forces)
    F_r = -V.zeta_a*v_measured^2 - V.c_r*V.m*V.g*cos(theta) - V.m*V.g*sin(theta); 

    % Required force
    F_t_req = V.m*V.lambda*a_opt - F_r;

    % Calculate rear wheel traction limit and total traction limit
    F_f_r_max = V.mu/V.L*( V.m*V.g*( V.L_f*cos(theta) + V.h_g*sin(theta) ) + V.h_g*( V.zeta_a*v_measured^2 + V.lambda*V.m*a_opt ) );
    F_f_tot_max = V.mu*V.m*V.g*cos(theta);

    % Correct for traction force (friction) and motor limits (torque)
    if F_t_req < 0 
        % braking
        if v_measured < V.omega_m_r/V.phi
            F_m_min = -V.phi*V.T_m_max/V.eta_TF;
        else
            F_m_min = -V.P_m_max/V.eta_TF/v_measured;
        end
        Fm_opt = max([F_t_req,F_m_min,-F_f_r_max]);
        Fb_opt = max(F_t_req,-F_f_tot_max) - Fm_opt;
    else
        % propulsion
        if v_measured < V.omega_m_r/V.phi
            F_m_max = V.phi*V.T_m_max*V.eta_TF;
        else
            F_m_max = V.P_m_max*V.eta_TF/v_measured;
        end
        Fm_opt = min([F_t_req,F_m_max,F_f_r_max]);
        Fb_opt = 0;
    end
    
    % Get the 'corrected' acceleration
    a_opt = (Fm_opt + Fb_opt + F_r)/V.m/V.lambda; % realized acceleration

    % Calculate other optimal quantities
    % cost  = full(sol.cost);
    % tLoop = toc(tLoopTic);
    t_0 = t_0 + Ts;

end

== matlab function ACCMPC/Low Level Controller and Plant/Plant ==
  settings: updateMethod=DISCRETE
  data: v input; u input; dv output; RG input; act_gear output
function [dv, act_gear]  = vehFcn(v, u, RG)
%vehFcn  ODE file representing the dynamics of the longitudinal speed.

% use: [t,v] = ode45(@(t,v) vehFcn(t, v, u, theta), tspan, v0);  % One comma removed
persistent m Tm wm Beta a_n gear  g
 if isempty(m)
     m       = 3283;     % kg mass
     g       = 9.8;      % m/s2
     Tm      = 390;      % Nm
     wm      = 418.8790; % rad/s (about 4000 RPM),;      % rad/s (about 4000 RPM),
     Beta    = 0.4;      % 
     %r      = 0.6;      % m - loaded wheel radious
     a_n     = [47.2 33.2 21.1 16.7 12.9 10.0 8.4 6.7]'; 

     % variables updated internaly:
     gear    = 1;
 end

theta = atan(RG/100);
%% intermediate eqs:
% gear selection:
if v <= 6  
   gear = 1;  
elseif v > 6 && v <= 10 
   gear = 2;
elseif v > 10 && v <= 13
   gear = 3;
elseif v > 13 && v <= 18
   gear = 4;
elseif v > 18 && v <= 24
   gear = 5;
elseif v > 24 && v <= 33
   gear = 6;
elseif v > 33 && v <= 41
   gear = 7;  
elseif v > 41
   gear = 8;  
end

% engine speed:
w = a_n(gear)*v;
% w = n/r*v

% engine torque:
Te = Tm*(1 - Beta*(w/wm-1)^2);

F0 = 345;
F1 = 0;
F2 = 0.1007/(1/3.6)^2;

% gravity force:
Fg = m*g*sin(theta);

% State equations.
dv = 1/m*(a_n(gear)*u*Te - F0 - F1*v - F2*v^2 - Fg); 
act_gear = gear;

== matlab function ACCMPC/Low Level Controller and Plant/FF Acceleration LUIS/FEEDFORWARD ==
  settings: updateMethod=DISCRETE
  data: acc_target input; v_ref input; uff output; RG input; gear input
function uff  = feedforward(acc_target, v_ref, RG, gear)
%FEEDFORWARD Summary of this function goes here
%   Detailed explanation goes here

persistent m Te_max w_max beta a_n F0 F1 F2 a_n_all g
 if isempty(m)
     m          = 3283;     % kg mass
     g          = 9.8;      % m/s2
     Te_max     = 390;      % Nm
     w_max      = 418.8790; % rad/s (about 4000 RPM),
     beta       = 0.4;      % 
     %r        = 0.6;      % m - loaded wheel radious

     % w_eng = a_n(gear)*v: a_n(1) = 40; a_n(2) = 25; etc...
     a_n_all = [47.2 33.2 21.1 16.7 12.9 10.0 8.4 6.7]';

     F0 = 345;
     F1 = 0;
     F2 = 0.1007/(1/3.6)^2;

 end
theta = atan(RG/100);
%% intermediate eqs:
a_n = a_n_all(gear);

dvdt = acc_target;
uff = -(m*(dvdt + (F2*v_ref^2 + F1*v_ref + F0 + g*m*sin(theta))/m))/(Te_max*a_n*(beta*((a_n*v_ref)/w_max - 1)^2 - 1));
end

== matlab function ACCMPC/Low Level Controller and Plant/FF_Braking/Braking_FEEDFORWARD ==
  settings: updateMethod=DISCRETE
  data: acc_target input; v input; theta_FF output; gear input; RG input
function theta_FF  = feedforward(acc_target, v, gear, RG)
%FEEDFORWARD Summary of this function goes here
%   Detailed explanation goes here
theta = atan(RG/100); 

persistent m F0 F1 F2 a_n_all g
 if isempty(m)
     m          = 3283;     % kg mass
     g          = 9.8;      % m/s2
     Te_max     = 390;      % Nm
     w_max      = 418.8790; % rad/s (about 4000 RPM),
     beta       = 0.4;      % 
     %r        = 0.6;      % m - loaded wheel radious

     % w_eng = a_n(gear)*v: a_n(1) = 40; a_n(2) = 25; etc...
     a_n_all = [47.2 33.2 21.1 16.7 12.9 10.0 8.4 6.7]';

     F0 = 345;
     F1 = 0;
     F2 = 0.1007/(1/3.6)^2;

 end

%% intermediate eqs:
a_n = a_n_all(gear);

dvdt = acc_target;

theta_FF = max(0,-theta - asin((F0 + F1*v + dvdt*m + F2*v^2)/(g*m)));

end
